simulink model "pandO_matlab_Final"  (R2020a)
settings: Solver=ode23tb  StartTime=0.0  StopTime=0.1  RelTol=1e-3
undefined symbols (not defined in the file or in its folder): sigbuilder_block
libraries: powerlib x8, powerlib_meascontrol x1, re_lib x1
settings Model: Creator=Rodney Tan  LastModifiedBy=sameeraa
settings SolverCC: ZeroCrossAlgorithm=Adaptive
settings DataIOCC: ReturnWorkspaceOutputs=off
settings DebuggingCC: MaxConsecutiveZCsMsg=none  MaskedZcDiagnostic=none  IgnoredZcDiagnostic=none  ArithmeticOperatorsInVariantConditions=warning
settings SFSimCC: SimUseLocalCustomCode=off  CustomCodeUndefinedFunction=UseInterfaceOnly
settings RTWCC: RTWUseLocalCustomCode=off

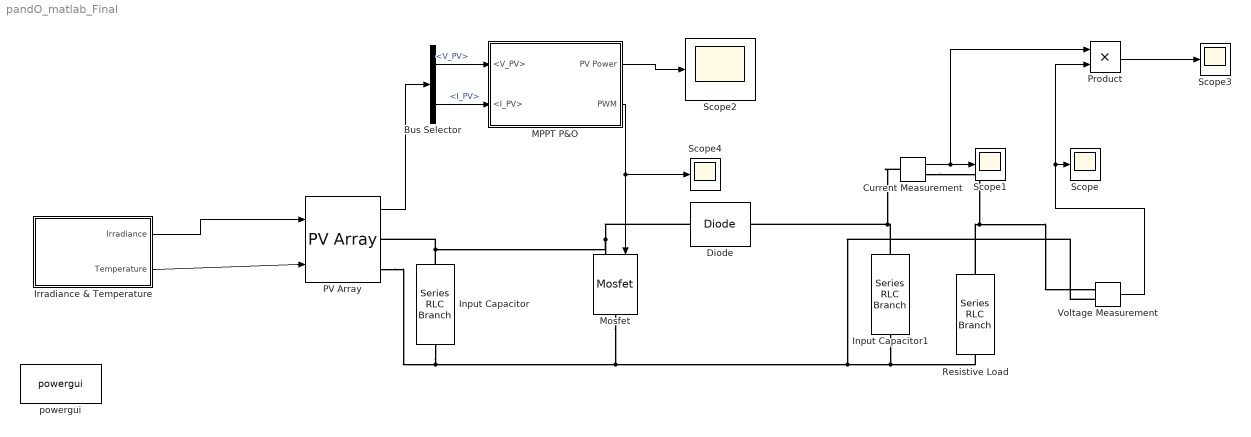
== system pandO_matlab_Final ==
  Bus Selector : BusSelector  OutputSignals=V_PV,I_PV
  Current Measurement : powerlib/Measurements/Current Measurement  PhasorSimulation=off  OutputType=Complex  PSBequivalent=0
  Diode : powerlib/Power Electronics/Diode  Ron=0.001  Lon=0  Vf=0.8  IC=0  UseSnubber=0  Rs=500  Cs=250e-9  Measurements=off
  Input Capacitor : powerlib/Elements/Series RLC Branch  LConnTagsString=__new0  RConnTagsString=__new0  BranchType=C  Resistance=10  Inductance=1e-3  SetiL0=off  InitialCurrent=0  Capacitance=1000e-6  Setx0=off  InitialVoltage=0  Measurements=None
  Input Capacitor1 : powerlib/Elements/Series RLC Branch  LConnTagsString=__new0  RConnTagsString=__new0  BranchType=C  Resistance=10  Inductance=1e-3  SetiL0=off  InitialCurrent=0  Capacitance=3777e-6  Setx0=off  InitialVoltage=0  Measurements=None
  Irradiance & Temperature : Subsystem  Tag=STV Subsys  LoadFcn=sigbuilder_block('load');  StartFcn=sigbuilder_block('start');  StopFcn=sigbuilder_block('stop');  ClipboardFcn=sigbuilder_block('clipboard');  mask(Sigbuilder block){tuvar=[0:10]}
      mask help: Simulink:masks:SigbuilderBlock_MD
      mask init:
      | if ~strcmp(get_param(bdroot(gcbh),'SimulationStatus'),'stopped') tuvar = sigbuilder_block('maskInit'); end
      settings: CopyFcn=sigbuilder_block('copy');  DeleteFcn=sigbuilder_block('delete');  ModelCloseFcn=sigbuilder_block('modelClose');  PreSaveFcn=sigbuilder_block('preSave');  PauseFcn=sigbuilder_block('pause');  ContinueFcn=sigbuilder_block('continue');  NameChangeFcn=sigbuilder_block('namechange');  OpenFcn=sigbuilder_block('open',[382.8 123 550.8 400.2 ]);  CloseFcn=sigbuilder_block('close');
      mask Display: plot(0, 0, 100, 100,[2, 2, 32, 32, 2], [68, 8, 8, 68, 68],[32, 2], [38, 38], [32, 19, 2],[53, 60, 44], [32, 17, 17, 2],[16, 16, 31, 31]);txt = getActiveGroup(gcbh);text(2, 100, txt,'verticalAlignment', 'top');
  "MPPT P&O " : Subsystem  mask(MPPT Perturbation & Observation Block){Fsw=10e3, StepSize=0.33}
      mask prompts: Fsw "PWM Switching frequency (Hz):"; StepSize "PWM Duty Cycle (delta) Step Size"
      mask help:
      | MPPT Perturbation & Observation Block
      | Developed by Rodney Tan (PhD)
      | Version 1.00 Aug 2019
      |
      | This block perform photovoltiac panel Maximum Power Point Tracking based on Perturbation & Observation algorithm.
      | This MPPT P&O method is implemented using MATLAB code scripted in MATLAB function block.
      | This MPPT block take in Voltage and Current from photovoltaic panel and output PWM switching signal to drive DC converter
      mask Help:
      | <b><u>Block Setting</u></b>
      | <b>PWM Switching Frequency (Hz)</b>
      | Specify the PWM switching frequency in Hz.
      | 
      | <b>PWM Duty Cycle Step Size</b>
      | Specify the PWM duty cycle (delta) step size. Default value is 1e-5.
      mask TypeOptions Fsw:
      | PWM Generator
      | (DC-DC)/Fsw
  Mosfet : powerlib/Power Electronics/Mosfet  Ron=0.1  Lon=0  Rd=0.01  Vfd=0  IC=0  Rs=1e5  Cs=inf  Measurements=off
  PV Array : re_lib/Solar/PV Array  Npar=40  Nser=5  PlotType=array @ 1000 W/m2 & specified temperatures  S_vec="[ 1000  500  100 ]"  Temp_C_vec="[ 45 25  ]"  ModuleName=1Soltech 1STH-250-WH  PlotWhenSelected=off  Pm=250.205  Ncell=60  Voc=37.3  Isc=8.66  Vm=30.7  Im=8.15  beta_Voc_pc=-0.36901  alpha_Isc_pc=0.086998  beta_Voc=-0.13764  alpha_Isc=0.007534  IL=8.7106  I0=4.1601e-10  nI=1.019  Rsh=224.1886  Rs=0.23724  RobustModel=off  RobustCellTemperature=25  BAL=on  Tc=1e-6  Tfilter=5e-5
  Product : Product
  Resistive Load : powerlib/Elements/Series RLC Branch  LConnTagsString=__new0  RConnTagsString=__new0  BranchType=R  Resistance=5  Inductance=1e-3  SetiL0=off  InitialCurrent=0  Capacitance=1e-6  Setx0=off  InitialVoltage=0  Measurements=None
  Scope{,1..4} (5 alike) : Scope
  Voltage Measurement : powerlib/Measurements/Voltage Measurement  PhasorSimulation=off  OutputType=Complex  PSBequivalent=0
  powergui : powerlib/powergui  Priority=1  SimulationMode=Continuous  SampleTime=1e-5  frequency=60  Iterations=50  frequencyindice=0  Pbase=100e6  ErrMax=1e-4  UnitsV=kV  UnitsW=MW  buscounter=0  FunctionMessages=off  echomessages=off  EnableUseOfTLC=off  CurrentSourceSwitches=off  DisableSnubberDevices=off  DisableRonSwitches=off  DisableVfSwitches=off  DisplayEquations=off  AutomaticDiscreteSolvers=off  SolverType=Tustin/Backward Euler (TBE)  Interpol=off  ExternalGateDelay=off  methode=off  Ts=100  x0status=blocks  SPID=off  SwTol=0  HookPort=off  NonlinearTolerance=1e-4  nMaxIteration=100  ContinueOnMaxIteration=off  RestoreLinks=warning  ResistiveCurrentMeasurement=off  Frange=[0:2:500]  Ylog=off  Xlog=on  ShowGrid=off  save=off  variable=ZData  structure=0  ZoomFFT=off  StartTime=0.0  cycles=1  DisplayStyle=1  fundamental=60  FreqAxis=off  MaxFrequency=1000  frequencyindicesteady=1  RmsSteady=1  display=off
  wires:
  PV Array/1 -> Bus Selector/1
  "MPPT P&O "/2(PWM) -> Mosfet/1, Scope4/1
  Bus Selector/1 -> "MPPT P&O "/1(<V_PV>)  "<V_PV>"
  Bus Selector/2 -> "MPPT P&O "/2(<I_PV>)  "<I_PV>"
  "MPPT P&O "/1(PV Power) -> Scope2/1
  Voltage Measurement/1 -> Product/2, Scope/1
  Current Measurement/1 -> Product/1, Scope1/1
  Irradiance & Temperature/1(Irradiance) -> PV Array/1
  Irradiance & Temperature/2(Temperature) -> PV Array/2
  Product/1 -> Scope3/1
  connections:
  PV Array/RConn2 -- Mosfet/RConn1 -- Resistive Load/RConn1 -- Input Capacitor1/RConn1 -- Voltage Measurement/LConn2 -- Input Capacitor/RConn1
  Input Capacitor/LConn1 -- Diode/LConn1 -- Mosfet/LConn1 -- PV Array/RConn1
  Input Capacitor1/LConn1 -- Current Measurement/LConn1 -- Diode/RConn1
  Resistive Load/LConn1 -- Current Measurement/RConn1 -- Voltage Measurement/LConn1

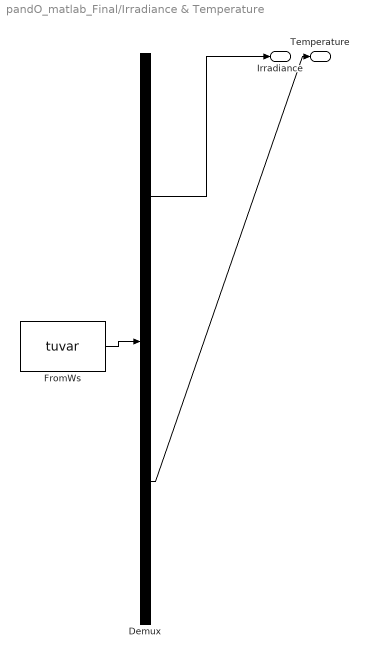
== system pandO_matlab_Final/Irradiance & Temperature ==
  Demux : Demux  Tag=STV Demux  Outputs=2
      settings: DisplayOption=none
  FromWs : FromWorkspace  Tag=STV FromWs  VariableName=tuvar
      SigBuilderData=|
      | common.afterFinalStr = 'Extrapolate'
      | common.sampleTime = 0
      | dataSet.timeRange = [0 10]
      | dataSet.name = 'Group 1'
      | sbobj.Groups.Name = 'Group 1'
      | sbobj.Groups.Signals(1).Name = 'Irradiance'
      | sbobj.Groups.Signals(1).XData = [0 10]
      | sbobj.Groups.Signals(1).YData = [1000 1000]
      | sbobj.Groups.Signals(2).Name = 'Temperature'
      | sbobj.Groups.Signals(2).XData = [0 10]
      | sbobj.Groups.Signals(2).YData = [25 25]
  Irradiance : Outport  Tag=STV Outport
  Temperature : Outport  Tag=STV Outport  Port=2
  wires:
  Demux/1 -> Irradiance/1
  FromWs/1 -> Demux/1
  Demux/2 -> Temperature/1

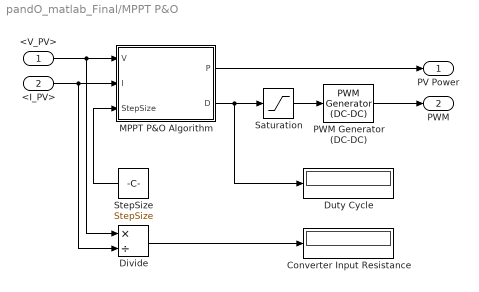
== system pandO_matlab_Final/MPPT P&O  ==
  <V_PV> : Inport
  <I_PV> : Inport  Port=2
  Converter Input Resistance : Display
  Divide : Product  Inputs=*/
  Duty Cycle : Display
  MPPT P&O Algorithm : MATLAB Function  TreatAsAtomicUnit=on
  PWM Generator (DC-DC) : powerlib_meascontrol/Pulse & Signal Generators/PWM Generator (DC-DC)  Fsw=Fsw  Ts=0
  Saturation : Saturate  UpperLimit=1  LowerLimit=0
  StepSize : Constant  Value=StepSize
  PV Power : Outport  VectorParamsAs1DForOutWhenUnconnected=off
  PWM : Outport  Port=2  VectorParamsAs1DForOutWhenUnconnected=off
  wires:
  <I_PV>/1 -> MPPT P&O Algorithm/2(I), Divide/2
  <V_PV>/1 -> MPPT P&O Algorithm/1(V), Divide/1
  PWM Generator (DC-DC)/1 -> PWM/1
  Divide/1 -> Converter Input Resistance/1
  Saturation/1 -> PWM Generator (DC-DC)/1
  MPPT P&O Algorithm/1(P) -> PV Power/1
  MPPT P&O Algorithm/2(D) -> Saturation/1, Duty Cycle/1
  StepSize/1 -> MPPT P&O Algorithm/3(StepSize)

== matlab function pandO_matlab_Final/MPPT P&O /MPPT P&O Algorithm ==
  settings: updateMethod=DISCRETE
  data: P output; V input; D output; I input; StepSize input
function [P, D] = fcn(V,I,StepSize)
    % Initialization
    persistent Pprev Vprev Dprev
    if isempty(Pprev)
        Pprev = 0;
        Vprev = 0;
        Dprev = 0.5;
    end
    % P&O Algorithm Begin here
    P = I*V;
    if (P-Pprev) > 0
        if (V-Vprev) > 0
            D = Dprev - StepSize;
        else
            D = Dprev + StepSize;
        end
    else
        if (V-Vprev) > 0
            D = Dprev + StepSize;
        else
            D = Dprev - StepSize;
        end
    end
    % Update current value to previous value
    Pprev = P;
    Vprev = V;
    Dprev = D;
end
